simulink model "observador_de_estado"  (R2023b)
settings: Solver=VariableStepAuto  StartTime=0.0  StopTime=10.0  RelTol=1e-3
values from neighbouring files (symbols this model uses):
  Jeq_nom = Jm + Jl_nom/r^2    (= 1.97847222222e-05)    [params_subsistema_mecanico.m]    (also in sistema_completo_en_codigo.m)
settings Model: Creator=Pc  LastModifiedBy=Pc

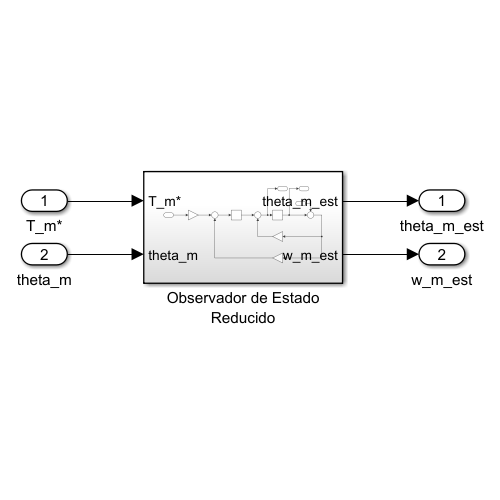
[thumbnail: Simulink's stored preview of the top-level diagram]
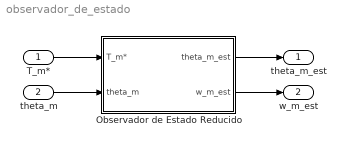
== system observador_de_estado ==
  T_m* : Inport
  theta_m : Inport  Port=2
  Observador de Estado Reducido : Subsystem
  theta_m_est : Outport
  w_m_est : Outport  Port=2
  wires:
  T_m*/1 -> Observador de Estado Reducido/1(T_m*)
  theta_m/1 -> Observador de Estado Reducido/2(theta_m)
  Observador de Estado Reducido/2(w_m_est) -> w_m_est/1
  Observador de Estado Reducido/1(theta_m_est) -> theta_m_est/1

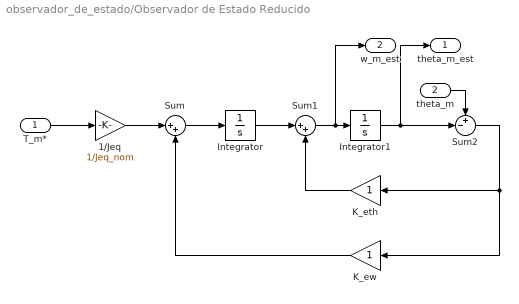
== system observador_de_estado/Observador de Estado Reducido ==
  T_m* : Inport
  theta_m : Inport  Port=2
  1/Jeq : Gain  Gain=1/Jeq_nom
  Integrator : Integrator
  Integrator1 : Integrator
  K_eth : Gain
  K_ew : Gain
  Sum : Sum  Inputs=|++
  Sum1 : Sum  Inputs=|++
  Sum2 : Sum  Inputs=+-|
  theta_m_est : Outport
  w_m_est : Outport  Port=2
  wires:
  Integrator1/1 -> theta_m_est/1, Sum2/2
  Sum2/1 -> K_eth/1, K_ew/1
  Sum1/1 -> w_m_est/1, Integrator1/1
  theta_m/1 -> Sum2/1
  K_eth/1 -> Sum1/2
  Sum/1 -> Integrator/1
  1/Jeq/1 -> Sum/1
  K_ew/1 -> Sum/2
  T_m*/1 -> 1/Jeq/1
  Integrator/1 -> Sum1/1
